simulink model "example5"  (Simulink 7.1)
settings: Solver=ode45  StartTime=0.0  StopTime=Tstop  MaxStep=intg_maxstep  RelTol=1e-6
model workspace: external: M-Code (data not in the file)
undefined symbols (not defined in the file or in its folder): q_init, x_init
libraries: simulink x1
settings Model: Creator=roy  LastModifiedBy=roy
settings DataIOCC: LimitDataPoints=off

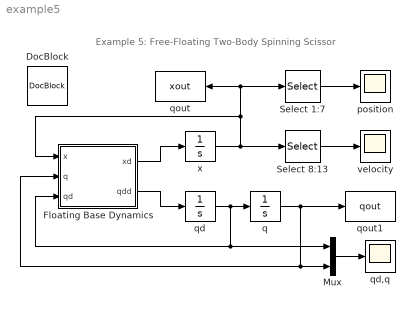
== system example5 ==
  note: Example 5: Free-Floating Two-Body Spinning Scissor
  DocBlock : simulink/Model-Wide Utilities/DocBlock  SystemSampleTime=-1  DocumentType=Text
      content=|
      | This example shows how to use the function FDfb on a system that contains
      | both a floating base and one or more real joints.  In this case, the
      | system is a pair of identical rectangular bodies that are connected at the
      | middle by a revolute joint, making a scissor-like mechanism.
      |
      | The problem that must be solved is this: FDfb returns two vectors, xd and
      | qdd, but a "Matlab Function" block in Simulink expects only a single
      | return value.  In Example 4 the problem did not arise because qdd was an
      | empty matrix (because there were no joints in that system other than the
      | six making the floating base).  The solution shown in this example is to
      | use a wrapper function, gcFD, that acts as an interface between Simulink
      | and several forward-dynamics functions, including FDfb.
      |
      | If you open the block "FDfb wrapper", which is inside the subsystem
      | "Floating Base Dynamics", you will find that the function call is
      | "gcFD(scissor,@FDfb,u)".  You will also see that the output dimensions
      | are 14x1.  This function (which you can find in the simulink subdirectory)
      | splits u into its component parts (x, q, qd, etc.), calls FDfb,
      | concatenates its two return values into a single vector, and returns it.
      | As scissor has only a single real joint, the dimensions of xd and qdd will
      | be 13x1 and 1x1, respectively, and so the dimension of the vector returned
      | by gcFD is 14x1.  This vector is then immediately split into its component
      | parts by the demultiplexor block.  The expression @FDfb is a Matlab
      | function handle.  It tells gcFD which forward-dynamics function to use.
      |
      | Having solved the problem of getting two outputs from FDfb, all that
      | remains to be done is to integrate these outputs and feed the results back
      | into the dynamics calculation block.  xd only needs to be integrated once,
      | and then fed back to the input "x" in the dynamics block; but qdd needs to
      | be integrated twice, and the two results fed back into the inputs labelled
      | "qd" and "q".  The rest of this Simulink model displays x in two scopes
      | (one for position variables and the other for velocity variables), and
      | displays q and qd together in a single scope.  It also saves q and x to
      | the Matlab workspace variables qout and xout.
      |
      | This simulation is ready to go.  Just click "Start", and watch the signals
      | appear on the scopes.  The resulting curves look interesting, but are a
      | bit difficult to interpret.  The motion is easier to understand if you see
      | it in showmotion.  The command to do this is
      | "showmotion(scissor,tout,fbanim(xout,qout))".  (Observe that fbanim now
      | takes two arguments, compared with only one in Example 4.)  The motion
      | should now make sense.
      |
      | If you want to try modifying the initial conditions, then fire up the
      | model explorer and take a look at the model workspace of Example 5.  There
      | you will find the Matlab code that determines the initial conditions.  The
      | two variables of interest are q_init, which determines the initial opening
      | of the two scissor blades, and w_init, which determines the initial
      | angular velocity of the mechanism.  If you decide to change them, remember
      | that you have to click "Apply" and then click "Reinitialize from Source"
      | before the changes take effect.
  Floating Base Dynamics : Subsystem
  Mux : Mux  Inputs=2
  Select 1:7 : Selector  InputPortWidth=13  IndexOptions=Index vector (dialog)  Indices=[1 2 3 4 5 6 7]  OutputSizes=1
  Select 8:13 : Selector  InputPortWidth=13  IndexOptions=Index vector (dialog)  Indices=[8 9 10 11 12 13]  OutputSizes=1
  position : Scope
      settings: YMin=-1.5  YMax=1.5
  q : Integrator  InitialCondition=q_init
  qd : Integrator
  qd,q : Scope
      settings: YMin=-2  YMax=7  SaveName=ScopeData2
  qout : ToWorkspace  VariableName=xout  SampleTime=-1  SaveFormat=Array
  qout1 : ToWorkspace  VariableName=qout  SampleTime=-1  SaveFormat=Array
  velocity : Scope
      settings: YMin=-2  YMax=4
  x : Integrator  InitialCondition=x_init
  wires:
  Floating Base Dynamics/1(xd) -> x/1
  Select 1:7/1 -> position/1
  Select 8:13/1 -> velocity/1
  Floating Base Dynamics/2(qdd) -> qd/1
  x/1 -> Select 8:13/1, Floating Base Dynamics/1(x), Select 1:7/1, qout/1
  q/1 -> qout1/1, Floating Base Dynamics/2(q), Mux/2
  Mux/1 -> qd,q/1
  qd/1 -> q/1, Mux/1, Floating Base Dynamics/3(qd)

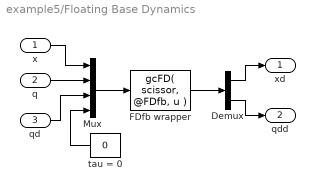
== system example5/Floating Base Dynamics ==
  x : Inport  OutDataType=sfix(16)  OutScaling=2^0
  q : Inport  Port=2  OutDataType=sfix(16)  OutScaling=2^0
  qd : Inport  Port=3  OutDataType=sfix(16)  OutScaling=2^0
  Demux : Demux  Outputs=[13 1]
  FDfb wrapper : MATLABFcn  MATLABFcn=gcFD( scissor, @FDfb, u )  OutputDimensions=[14 1]  OutputSignalType=real  Output1D=off
  Mux : Mux
  tau = 0 : Constant  Orientation=left  Value=0  OutDataType=sfix(16)  OutScaling=2^0
  xd : Outport  OutDataType=sfix(16)  OutScaling=2^0
  qdd : Outport  Port=2  OutDataType=sfix(16)  OutScaling=2^0
  wires:
  Mux/1 -> FDfb wrapper/1
  FDfb wrapper/1 -> Demux/1
  Demux/1 -> xd/1
  Demux/2 -> qdd/1
  q/1 -> Mux/2
  qd/1 -> Mux/3
  x/1 -> Mux/1
  tau = 0/1 -> Mux/4
